simulink model "Lumped_parameter_sim"  (R2019a)
settings: Solver=ode15s  StartTime=0.0  StopTime=s_time  MaxStep=h  RelTol=1e-6
values from neighbouring files (symbols this model uses):
  R_in = 0.1108    [Main.m]
  R_out = 0.1108    [Main.m]
libraries: fl_lib x15, ee_lib x6, nesl_utility x5, simulink x2
settings Model: Creator=mpmci  LastModifiedBy=mpmci

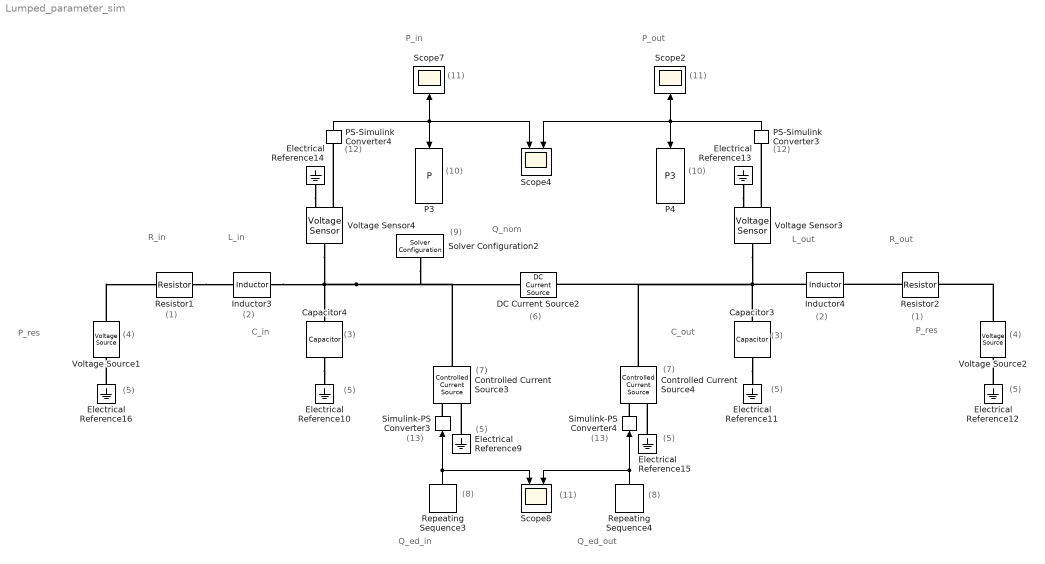
== system Lumped_parameter_sim ==
  note: (3)
  note: L_in
  note: (5)
  note: R_in
  note: C_in
  note: (4)
  note: (1)
  note: (5)
  note: Q_ed_out
  note: R_out
  note: P_in
  note: C_out
  note: (5)
  note: (3)
  note: Q_ed_in
  note: (2)
  note: L_out
  note: (2)
  note: (1)
  note: (6)
  note: (7)
  note: (8)
  note: Q_nom
  note: (11)
  note: P_res
  note: (12)
  note: (12)
  note: (5)
  note: (13)
  note: (4)
  note: (7)
  note: (9)
  note: (11)
  note: (10)
  note: (8)
  note: (5)
  note: (13)
  note: (11)
  note: P_res
  note: (5)
  note: (10)
  note: P_out
  Capacitor3 : ee_lib/Passive/Capacitor  enable_table=0  c=C_out F  Cvec=[1e-05, 1e-06] F  Vvec=[0, 10] V  CV_table_symmetry=1  C_tol=5  enable_C_tol=0  tol_distribution=1  nSigma=4  r=1e-6 Ohm  g=0 1/Ohm  enable_operating_limits=0  operating_limit_action=2  max_working_voltage_range=[-25, 25] V  power_rating=1 W  enable_faults=0  fault_action=1  Cscale_faulted=100  R_faulted=1e-3 Ohm  G_faulted=0 1/Ohm  tau_fault=1e-3 s  enable_temporal_fault=0  t_fault=1 s  enable_behavioral_fault=0  max_permissible_voltage_range=[-100, 100] V  t_fail_on_voltage=1 s  i_specify=off  i_priority=None  i=0 A  i_nominal_specify=off  i_nominal_unit=A  i_nominal_value=1  v_specify=off  v_priority=None  v=0 V  v_nominal_specify=off  v_nominal_unit=V  v_nominal_value=1  vc_specify=off  vc_priority=High  vc=0 V  vc_nominal_specify=off  vc_nominal_unit=V  vc_nominal_value=1
      settings: SourceProductName=Simscape Electrical
  Capacitor4 : ee_lib/Passive/Capacitor  enable_table=0  c=C_in F  Cvec=[1e-05, 1e-06] F  Vvec=[0, 10] V  CV_table_symmetry=1  C_tol=0  enable_C_tol=0  tol_distribution=1  nSigma=4  r=1e-6 Ohm  g=0 1/Ohm  enable_operating_limits=0  operating_limit_action=2  max_working_voltage_range=[-25, 25] V  power_rating=1 W  enable_faults=0  fault_action=1  Cscale_faulted=100  R_faulted=1e-3 Ohm  G_faulted=0 1/Ohm  tau_fault=1e-3 s  enable_temporal_fault=0  t_fault=1 s  enable_behavioral_fault=0  max_permissible_voltage_range=[-100, 100] V  t_fail_on_voltage=1 s  i_specify=off  i_priority=None  i=0 A  i_nominal_specify=off  i_nominal_unit=A  i_nominal_value=1  v_specify=off  v_priority=None  v=0 V  v_nominal_specify=off  v_nominal_unit=V  v_nominal_value=1  vc_specify=off  vc_priority=High  vc=0 V  vc_nominal_specify=off  vc_nominal_unit=V  vc_nominal_value=1
      settings: SourceProductName=Simscape Electrical
  Controlled Current Source3 : fl_lib/Electrical/Electrical Sources/Controlled Current Source
  Controlled Current Source4 : fl_lib/Electrical/Electrical Sources/Controlled Current Source
  DC Current Source2 : fl_lib/Electrical/Electrical Sources/DC Current Source  i0=Q_nom A
      settings: SourceProductName=Simscape  SourceProductBaseCode=SS
  Electrical Reference{9..16} (8 alike) : fl_lib/Electrical/Electrical Elements/Electrical Reference
  Inductor3 : ee_lib/Passive/Inductor  l=L_in H  L_tol=0  enable_L_tol=0  tol_distribution=1  nSigma=4  r=1e-9 Ohm  g=1e-9 1/Ohm  enable_operating_limits=0  operating_limit_action=2  max_working_current=1 A  power_rating=1 W  enable_faults=0  fault_action=1  lambdaPercent=50  k_faulted=0.9999  turnsShort=0  openCct=0  groundShort=0  groundShortG=0 1/Ohm  tau_fault=1e-3 s  enable_temporal_fault=0  t_fault=1 s  enable_behavioral_fault=0  max_permissible_voltage=100 V  n_fail_on_voltage=1  max_permissible_current=1 A  t_fail_on_current=1 s  i_L_specify=off  i_L_priority=High  i_L=0 A  i_L_nominal_specify=off  i_L_nominal_unit=A  i_L_nominal_value=1
      settings: SourceProductName=Simscape Electrical
  Inductor4 : ee_lib/Passive/Inductor  l=L_out H  L_tol=0  enable_L_tol=0  tol_distribution=1  nSigma=4  r=1e-9 Ohm  g=1e-9 1/Ohm  enable_operating_limits=0  operating_limit_action=2  max_working_current=1 A  power_rating=1 W  enable_faults=0  fault_action=1  lambdaPercent=50  k_faulted=0.9999  turnsShort=0  openCct=0  groundShort=0  groundShortG=0 1/Ohm  tau_fault=1e-3 s  enable_temporal_fault=0  t_fault=1 s  enable_behavioral_fault=0  max_permissible_voltage=100 V  n_fail_on_voltage=1  max_permissible_current=1 A  t_fail_on_current=1 s  i_L_specify=off  i_L_priority=High  i_L=0 A  i_L_nominal_specify=off  i_L_nominal_unit=A  i_L_nominal_value=1
      settings: SourceProductName=Simscape Electrical
  P3 : ToWorkspace  VariableName=P  SampleTime=-1
      settings: Save2DSignal=2-D array (concatenate along first dimension)
  P4 : ToWorkspace  VariableName=P3  SampleTime=-1
      settings: Save2DSignal=2-D array (concatenate along first dimension)
  PS-Simulink Converter3 : nesl_utility/PS-Simulink Converter  PhysicalDomain=network_engine_domain  SubClassName=ps_output  LeftPortType=input  RightPortType=output  PseudoPeriodic=off  Frequencies=[]  Unit=1  AffineConversion=off
  PS-Simulink Converter4 : nesl_utility/PS-Simulink Converter  PhysicalDomain=network_engine_domain  SubClassName=ps_output  LeftPortType=input  RightPortType=output  PseudoPeriodic=off  Frequencies=[]  Unit=1  AffineConversion=off
  Repeating Sequence3 : simulink/Sources/Repeating Sequence  rep_seq_t=t_vec  rep_seq_y=Q_ed_in
  Repeating Sequence4 : simulink/Sources/Repeating Sequence  rep_seq_t=t_vec  rep_seq_y=Q_ed_out
  Resistor1 : fl_lib/Electrical/Electrical Elements/Resistor  R=R_in Ohm  i_specify=off  i_priority=None  i=0 A  i_nominal_specify=off  i_nominal_unit=A  i_nominal_value=1  v_specify=off  v_priority=None  v=0 V  v_nominal_specify=off  v_nominal_unit=V  v_nominal_value=1
  Resistor2 : fl_lib/Electrical/Electrical Elements/Resistor  R=R_out Ohm  i_specify=off  i_priority=None  i=0 A  i_nominal_specify=off  i_nominal_unit=A  i_nominal_value=1  v_specify=off  v_priority=None  v=0 V  v_nominal_specify=off  v_nominal_unit=V  v_nominal_value=1
  Scope2 : Scope
  Scope4 : Scope  NumInputPorts=2
  Scope7 : Scope
  Scope8 : Scope  NumInputPorts=2
  Simulink-PS Converter3 : nesl_utility/Simulink-PS Converter  PhysicalDomain=network_engine_domain  SubClassName=ps_input  LeftPortType=input  RightPortType=output  PseudoPeriodic=off  Frequencies=[]  NoiseDistribution=none  NoiseParameters=[]  Unit=1  AffineConversion=off  FilteringAndDerivatives=provide  SimscapeFilterOrder=1  InputFilterTimeConstant=0.001  UdotUserProvided=0
  Simulink-PS Converter4 : nesl_utility/Simulink-PS Converter  PhysicalDomain=network_engine_domain  SubClassName=ps_input  LeftPortType=input  RightPortType=output  PseudoPeriodic=off  Frequencies=[]  NoiseDistribution=none  NoiseParameters=[]  Unit=1  AffineConversion=off  FilteringAndDerivatives=provide  SimscapeFilterOrder=1  InputFilterTimeConstant=0.001  UdotUserProvided=0
  Solver Configuration2 : nesl_utility/Solver Configuration  PhysicalDomain=network_engine_domain  SubClassName=solver  LeftPortType=input  RightPortType=generic  Tones=[]  Harmonics=[]  SimulateNoise=off  Profile=off  UseLocalSampling=off  EnableSwitchedLinearOptims=on  FrequencyDomain=off  UseCCode=off  RelTol=0.001  AbsTol=1e-06  MinStep=1e-09  ToWorkspace=off  RevertToSquareIcSolve=off  NumHomotopyIterations=100  PhasorMode=off  PhasorModeNumHarmonics=1  DoDC=off  ResidualTolerance=1e-09  UseLocalSolver=off  LocalSolverChoice=NE_BACKWARD_EULER_ADVANCER  LocalSolverSampleTime=0.001  DoFixedCost=off  MaxNonlinIter=3  MaxModeIter=2  LinearAlgebra=auto  EquationFormulation=NE_TIME_EF  DelaysMemoryBudget=1024  AutomaticFiltering=on  FilteringTimeConstant=0.001  PartitionStorageMethod=AS_NEEDED  PartitionMemoryBudget=1024  PartitionMethod=FAST
  Voltage Sensor3 : fl_lib/Electrical/Electrical Sensors/Voltage Sensor
  Voltage Sensor4 : fl_lib/Electrical/Electrical Sensors/Voltage Sensor
  Voltage Source1 : ee_lib/Sources/Voltage Source  dc_voltage=P_res V  ac_voltage=0 V  ac_shift=0 rad  ac_frequency=0 Hz  noise_mode=0  PSD=0 V^2/Hz  repeatability=1  auto_seed=162087197  user_seed=0  sample_time=1e-3 s  i_specify=off  i_priority=None  i=0 A  i_nominal_specify=off  i_nominal_unit=A  i_nominal_value=1  v_specify=off  v_priority=None  v=0 V  v_nominal_specify=off  v_nominal_unit=V  v_nominal_value=1
      settings: SourceProductName=Simscape Electrical
  Voltage Source2 : ee_lib/Sources/Voltage Source  dc_voltage=P_res V  ac_voltage=0 V  ac_shift=0 rad  ac_frequency=60 Hz  noise_mode=0  PSD=0 V^2/Hz  repeatability=1  auto_seed=3801767646  user_seed=0  sample_time=1e-3 s  i_specify=off  i_priority=None  i=0 A  i_nominal_specify=off  i_nominal_unit=A  i_nominal_value=1  v_specify=off  v_priority=None  v=0 V  v_nominal_specify=off  v_nominal_unit=V  v_nominal_value=1
      settings: SourceProductName=Simscape Electrical
  wires:
  PS-Simulink Converter4/1 -> Scope4/1, P3/1, Scope7/1
  PS-Simulink Converter3/1 -> Scope4/2, P4/1, Scope2/1
  Repeating Sequence3/1 -> Scope8/1, Simulink-PS Converter3/1
  Repeating Sequence4/1 -> Scope8/2, Simulink-PS Converter4/1
  connections:
  Voltage Sensor4/LConn1 -- Capacitor4/LConn1 -- Inductor3/RConn1 -- Controlled Current Source3/LConn1 -- DC Current Source2/RConn1 -- Solver Configuration2/RConn1
  Capacitor3/LConn1 -- DC Current Source2/LConn1 -- Controlled Current Source4/LConn1 -- Voltage Sensor3/LConn1 -- Inductor4/LConn1
  Voltage Source2/LConn1 -- Resistor2/RConn1
  Electrical Reference16/LConn1 -- Voltage Source1/RConn1
  Capacitor3/RConn1 -- Electrical Reference11/LConn1
  Electrical Reference12/LConn1 -- Voltage Source2/RConn1
  Capacitor4/RConn1 -- Electrical Reference10/LConn1
  Resistor1/RConn1 -- Inductor3/LConn1
  Voltage Sensor3/RConn1 -- PS-Simulink Converter3/LConn1
  Electrical Reference14/LConn1 -- Voltage Sensor4/RConn2
  Voltage Source1/LConn1 -- Resistor1/LConn1
  Simulink-PS Converter3/RConn1 -- Controlled Current Source3/RConn1
  Electrical Reference15/LConn1 -- Controlled Current Source4/RConn2
  Electrical Reference13/LConn1 -- Voltage Sensor3/RConn2
  Electrical Reference9/LConn1 -- Controlled Current Source3/RConn2
  Voltage Sensor4/RConn1 -- PS-Simulink Converter4/LConn1
  Simulink-PS Converter4/RConn1 -- Controlled Current Source4/RConn1
  Resistor2/LConn1 -- Inductor4/RConn1
